simulink model "Heaters_Bortoletto"  (R2025a)
settings: Solver=FixedStepAuto  StartTime=0.0  StopTime=600  FixedStep=1  RelTol=1e-3  EnableMultiTasking=on
InitFcn:
  | Tamb0 = 20;%°C
libraries: spsStairGeneratorLib x2
settings Model: Creator=johnh  LastModifiedBy=mocha
settings SolverCC: AlgebraicLoopSolver=TrustRegion
settings DataIOCC: ReturnWorkspaceOutputs=off
settings OptimizationCC: LifeSpan=inf
settings DebuggingCC: UnconnectedInputMsg=warning  UnconnectedOutputMsg=warning  UnconnectedLineMsg=warning  SFUnexpectedBacktrackingDiag=warning  SFNoUnconditionalDefaultTransitionDiag=warning  ArithmeticOperatorsInVariantConditions=warning
settings ModelReferenceCC: EnableRefExpFcnMdlSchedulingChecks=on
settings SFSimCC: SimUseLocalCustomCode=off  CustomCodeUndefinedFunction=UseInterfaceOnly
settings RTWCC: RTWUseLocalCustomCode=off  GPUComputeCapability=3.5
settings CodeAppCC: StateflowObjectComments=on
settings GRTTargetCC: TargetLangStandard=C89/C90 (ANSI)
settings ConfigComp: CovMetricSettings=dw  CovSaveCumulativeToWorkspaceVar=on  CovSaveSingleToWorkspaceVar=on  CovExternalEMLEnable=off

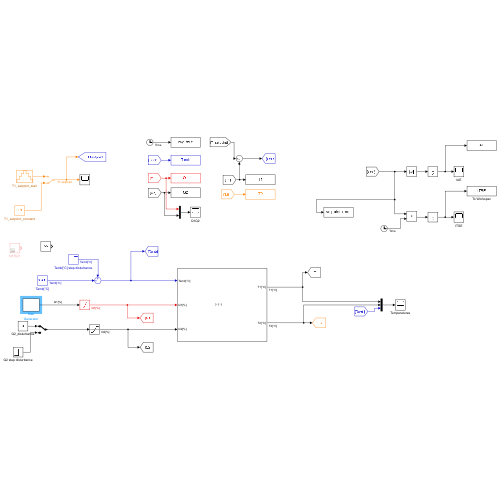
[thumbnail: Simulink's stored preview of the top-level diagram]
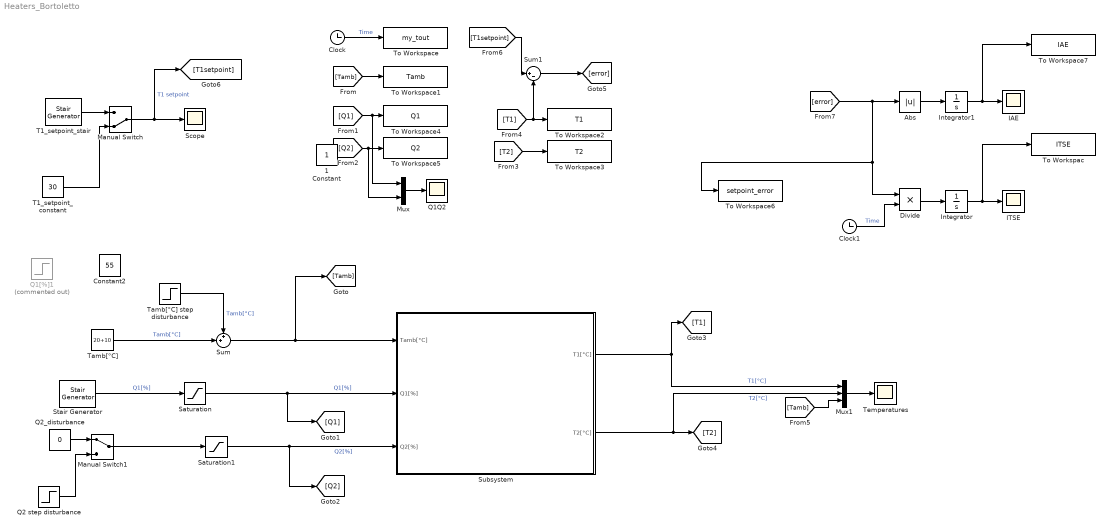
== system Heaters_Bortoletto ==
  Abs : Abs  SaturateOnIntegerOverflow=off
  Clock : Clock
  Clock1 : Clock
  Constant2 : Constant  Value=55
  Divide : Product  Inputs=**
  IAE : Scope
  ITSE : Scope
      settings: DataLoggingVariableName=ScopeData3
  Integrator : Integrator
  Integrator1 : Integrator
  Manual Switch : ManualSwitch  CurrentSetting=0
  Manual Switch1 : ManualSwitch
  Mux : Mux  Inputs=2
  Mux1 : Mux  Inputs=3
  Q1Q2 : Scope
      settings: ActiveDisplayYMinimum=-6.2499999999999982  ActiveDisplayYMaximum=56.25
  Q1[%]1 : Step  Commented=on  Time=0  After=80  SampleTime=0
  Q2 step disturbance : Step  Time=0  After=0  SampleTime=0
  Q2_disturbance : Constant  Value=0
  Saturation : Saturate  UpperLimit=100  LowerLimit=0
  Saturation1 : Saturate  UpperLimit=100  LowerLimit=0
  Scope : Scope
      settings: ActiveDisplayYMinimum=19.375  ActiveDisplayYMaximum=25.625  DataLoggingVariableName=ScopeData2
  Stair Generator : spsStairGeneratorLib/Stair Generator  t=[0, 300]  e=[50, 0]  Ts=0
  Subsystem : Subsystem
      mask Display: image('tclab.png');
  Sum : Sum  Inputs=++|
  Sum1 : Sum  Inputs=|+-
  T1_setpoint_constant : Constant  Value=30
  T1_setpoint_stair : spsStairGeneratorLib/Stair Generator  t=600*[0:8]  e=[20, 25, 30, 35, 40, 35, 30, 25, 20]  Ts=0
  Tamb[°C] : Constant  Value=20+10
  Tamb[°C] step disturbance : Step  Time=0  After=0  SampleTime=0
  Temperatures : Scope
      settings: ActiveDisplayYMinimum=2.8388394522749252  ActiveDisplayYMaximum=60.901685717525126
  To Workspac : ToWorkspace  VariableName=ITSE  SampleTime=-1
  To Workspace : ToWorkspace  VariableName=my_tout  SampleTime=-1
  To Workspace1 : ToWorkspace  VariableName=Tamb  SampleTime=-1
  To Workspace2 : ToWorkspace  VariableName=T1  SampleTime=-1
  To Workspace3 : ToWorkspace  VariableName=T2  SampleTime=-1
  To Workspace4 : ToWorkspace  VariableName=Q1  SampleTime=-1
  To Workspace5 : ToWorkspace  VariableName=Q2  SampleTime=-1
  To Workspace6 : ToWorkspace  VariableName=setpoint_error  SampleTime=-1
  To Workspace7 : ToWorkspace  VariableName=IAE  SampleTime=-1
  1 : Constant  IOType=siggen
  Constant : Constant  IOType=siggen
  wires:
  Subsystem/1(T1[°C]) -> Mux1/1, [T1]  "T1[°C]"
  Subsystem/2(T2[°C]) -> Mux1/2, [T2]  "T2[°C]"
  Saturation/1 -> Subsystem/2(Q1[%]), [Q1]  "Q1[%]"
  Saturation1/1 -> Subsystem/3(Q2[%]), [Q2]  "Q2[%]"
  Manual Switch1/1 -> Saturation1/1
  Tamb[°C]/1 -> Sum/2  "Tamb[°C]"
  Stair Generator/1 -> Saturation/1  "Q1[%]"
  Clock/1 -> To Workspace/1  "Time"
  [Tamb] -> To Workspace1/1
  [Q1] -> Mux/1, To Workspace4/1
  [Q2] -> Mux/2, To Workspace5/1
  [T2] -> To Workspace3/1
  [T1] -> Sum1/2, To Workspace2/1
  Mux1/1 -> Temperatures/1
  [Tamb] -> Mux1/3
  Mux/1 -> Q1Q2/1
  T1_setpoint_stair/1 -> Manual Switch/1
  T1_setpoint_constant/1 -> Manual Switch/2
  Manual Switch/1 -> [T1setpoint], Scope/1  "T1 setpoint"
  Divide/1 -> Integrator/1
  Clock1/1 -> Divide/2  "Time"
  Integrator/1 -> To Workspac/1, ITSE/1
  Q2_disturbance/1 -> Manual Switch1/1
  Q2 step disturbance/1 -> Manual Switch1/2
  Sum/1 -> Subsystem/1(Tamb[°C]), [Tamb]
  Tamb[°C] step disturbance/1 -> Sum/1  "Tamb[°C]"
  Abs/1 -> Integrator1/1
  Integrator1/1 -> To Workspace7/1, IAE/1
  [error] -> Divide/1, To Workspace6/1, Abs/1
  Sum1/1 -> [error]
  [T1setpoint] -> Sum1/1

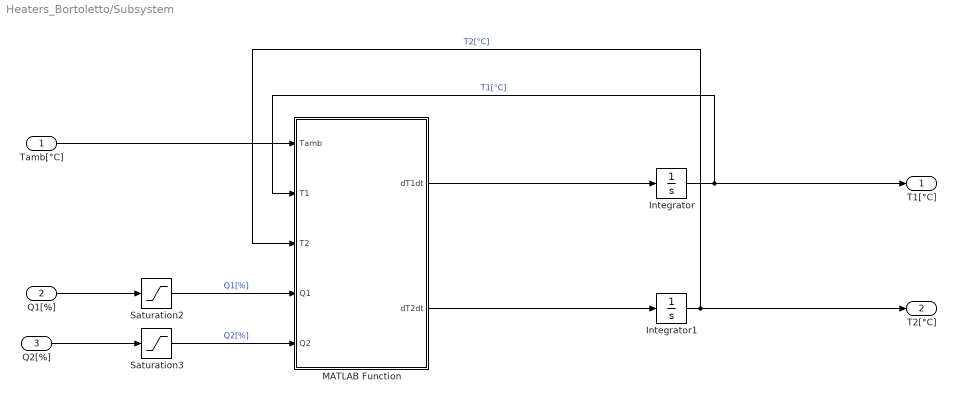
== system Heaters_Bortoletto/Subsystem ==
  Tamb[°C] : Inport
  Q1[%] : Inport  Port=2
  Q2[%] : Inport  Port=3
  Integrator : Integrator  InitialCondition=Tamb0
  Integrator1 : Integrator  InitialCondition=Tamb0
  MATLAB Function : MATLAB Function  TreatAsAtomicUnit=on
  Saturation2 : Saturate  UpperLimit=100  LowerLimit=0
  Saturation3 : Saturate  UpperLimit=100  LowerLimit=0
  T1[°C] : Outport
  T2[°C] : Outport  Port=2
  wires:
  Integrator1/1 -> T2[°C]/1, MATLAB Function/3(T2)  "T2[°C]"
  Integrator/1 -> T1[°C]/1, MATLAB Function/2(T1)  "T1[°C]"
  MATLAB Function/1(dT1dt) -> Integrator/1
  Saturation2/1 -> MATLAB Function/4(Q1)  "Q1[%]"
  Saturation3/1 -> MATLAB Function/5(Q2)  "Q2[%]"
  Q1[%]/1 -> Saturation2/1
  Q2[%]/1 -> Saturation3/1
  Tamb[°C]/1 -> MATLAB Function/1(Tamb)
  MATLAB Function/2(dT2dt) -> Integrator1/1

== matlab function Heaters_Bortoletto/Subsystem/MATLAB Function ==
  data: Tamb input; T1 input; dT1dt output; T2 input; Q1 input; Q2 input; dT2dt output
function [dT1dt, dT2dt] = arduino_ode(Tamb,T1,T2,Q1,Q2)
    % Parameters
    Ta = Tamb + 273.15;   % K
    U = 10.0;           % W/m^2-K
    m = 4.0/1000.0;     % kg
    Cp = 0.5 * 1000.0;  % J/kg-K    
    A = 10.0 / 100.0^2; % Area in m^2
    As = 2.0 / 100.0^2; % Area in m^2
    alpha1 = 0.0100;    % W / % heater 1
    alpha2 = 0.0075;    % W / % heater 2
    eps = 0.9;          % Emissivity
    sigma = 5.67e-8;    % Stefan-Boltzman

    % Temperature States 
    T1 = T1 + 273.15;   % K
    T2 = T2 + 273.15;   % K

    % Heat Transfer Exchange Between 1 and 2
    conv12 = sign(T2-T1)*U*As*(abs(T2-T1));
    rad12  = eps*sigma*As * (T2^4 - T1^4);

    % Nonlinear Energy Balances
    dT1dt = (1.0/(m*Cp))*(U*A*(Ta-T1) ...
            + eps * sigma * A * (Ta^4 - T1^4) ...
            + conv12 + rad12 ...
            + alpha1*Q1);
    dT2dt = (1.0/(m*Cp))*(U*A*(Ta-T2) ...
            + eps * sigma * A * (Ta^4 - T2^4) ...
            - conv12 - rad12 ...
            + alpha2*Q2);
end
